simulink model "Add6_Model"  (R2023a)
settings: Solver=VariableStepAuto  StartTime=0.0  StopTime=10.0  RelTol=1e-3
libraries: NSA_DEVS_SINKS_ATOMIC x7, NSA_DEVS_SOURCES_ATOMIC x6, NSA_DEVS_MATH_OPERATIONS_ATOMIC x1, NSA_DEVS_LOGISTICS_ATOMIC x1
settings Model: Creator=david  LastModifiedBy=david

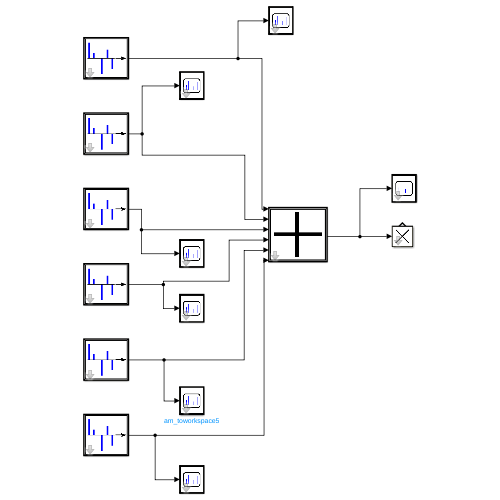
[thumbnail: Simulink's stored preview of the top-level diagram]
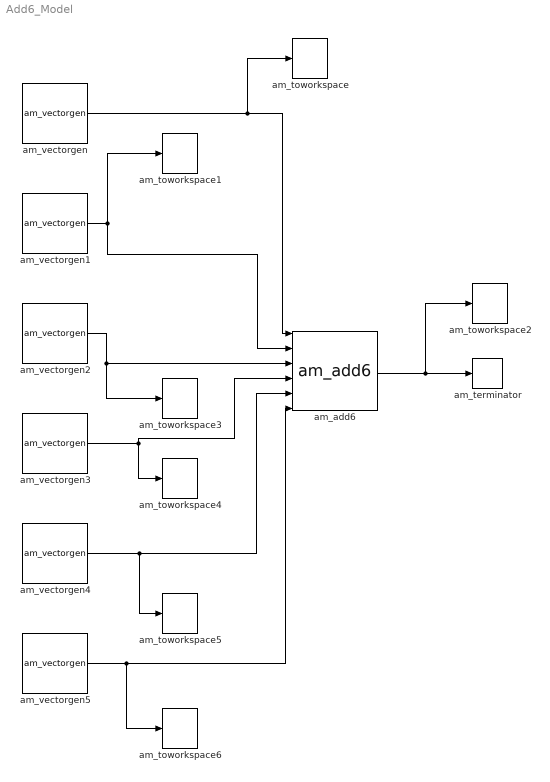
== system Add6_Model ==
  am_add6 : NSA_DEVS_MATH_OPERATIONS_ATOMIC/am_add6  tau=[0,1]  debug=0
      settings: SourceProductName=NSA_DEVS
  am_terminator : NSA_DEVS_LOGISTICS_ATOMIC/am_terminator  tau=[0,1]  debug=0
      settings: SourceProductName=NSA_DEVS
  am_toworkspace : NSA_DEVS_SINKS_ATOMIC/am_toworkspace  varname="\"gen1Out\""  t0=0  format="\"vector\""  tau=[0,5]  debug=0
      settings: SourceProductName=NSA_DEVS
  am_toworkspace1 : NSA_DEVS_SINKS_ATOMIC/am_toworkspace  varname="\"gen2Out\""  t0=0  format="\"vector\""  tau=[0,5]  debug=0
      settings: SourceProductName=NSA_DEVS
  am_toworkspace2 : NSA_DEVS_SINKS_ATOMIC/am_toworkspace  varname="\"addOut\""  t0=0  format="\"vector\""  tau=[0,5]  debug=0
      settings: SourceProductName=NSA_DEVS
  am_toworkspace3 : NSA_DEVS_SINKS_ATOMIC/am_toworkspace  varname="\"gen3Out\""  t0=0  format="\"vector\""  tau=[0,5]  debug=0
      settings: SourceProductName=NSA_DEVS
  am_toworkspace4 : NSA_DEVS_SINKS_ATOMIC/am_toworkspace  varname="\"gen4Out\""  t0=0  format="\"vector\""  tau=[0,5]  debug=0
      settings: SourceProductName=NSA_DEVS
  am_toworkspace5 : NSA_DEVS_SINKS_ATOMIC/am_toworkspace  varname="\"gen5Out\""  t0=0  format="\"vector\""  tau=[0,5]  debug=0
      settings: SourceProductName=NSA_DEVS
  am_toworkspace6 : NSA_DEVS_SINKS_ATOMIC/am_toworkspace  varname="\"gen6Out\""  t0=0  format="\"vector\""  tau=[0,5]  debug=0
      settings: SourceProductName=NSA_DEVS
  am_vectorgen : NSA_DEVS_SOURCES_ATOMIC/am_vectorgen  tvec=[1, 3, 5, 7, 9]  yvec=[2, 3, 2, 5, 7]  tau=[0,1]  debug=0
      settings: SourceProductName=NSA_DEVS
  am_vectorgen1 : NSA_DEVS_SOURCES_ATOMIC/am_vectorgen  tvec=[1, 3, 5, 7.3, 9.3]  yvec=[1, 2, 3, 6, 7]  tau=[0,1]  debug=0
      settings: SourceProductName=NSA_DEVS
  am_vectorgen2 : NSA_DEVS_SOURCES_ATOMIC/am_vectorgen  tvec=[1.5, 1.7, 5, 7, 9.1]  yvec="[3,   2.1, 6, 6, 5]"  tau=[0,1]  debug=0
      settings: SourceProductName=NSA_DEVS
  am_vectorgen3 : NSA_DEVS_SOURCES_ATOMIC/am_vectorgen  tvec=[1.5, 3.5, 5.5, 7.5, 9.5]  yvec=[2, 3, 2, 5, 7]  tau=[0,1]  debug=0
      settings: SourceProductName=NSA_DEVS
  am_vectorgen4 : NSA_DEVS_SOURCES_ATOMIC/am_vectorgen  tvec=[1.75, 3.75, 5.75, 7.75, 9.75]  yvec=[2, 3, 2, 5, 7]  tau=[0,1]  debug=0
      settings: SourceProductName=NSA_DEVS
  am_vectorgen5 : NSA_DEVS_SOURCES_ATOMIC/am_vectorgen  tvec=[1.8, 3.8, 5.8, 7.8, 9.8]  yvec=[2, 3, 2, 5, 7]  tau=[0,1]  debug=0
      settings: SourceProductName=NSA_DEVS
  wires:
  am_vectorgen/1 -> am_add6/1, am_toworkspace/1
  am_add6/1 -> am_toworkspace2/1, am_terminator/1
  am_vectorgen1/1 -> am_add6/2, am_toworkspace1/1
  am_vectorgen2/1 -> am_add6/3, am_toworkspace3/1
  am_vectorgen3/1 -> am_add6/4, am_toworkspace4/1
  am_vectorgen4/1 -> am_toworkspace5/1, am_add6/5
  am_vectorgen5/1 -> am_toworkspace6/1, am_add6/6
